simulink subsystem "ComputeState"  (R2020b)
settings: Solver=VariableStepAuto  StartTime=0.0  StopTime=10.0  RelTol=1e-3
libraries: simulink x2
settings Model: Creator=Marcus  LastModifiedBy=Marcus

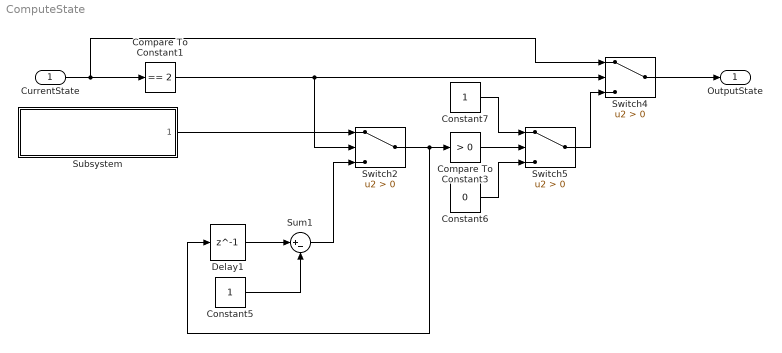
== system ComputeState ==
  CurrentState : Inport
  Compare To Constant1 : simulink/Logic and Bit Operations/Compare To Constant  relop===  const=2  OutDataTypeStr=boolean
  Compare To Constant3 : simulink/Logic and Bit Operations/Compare To Constant  relop=>  const=0  OutDataTypeStr=boolean
  Constant5 : Constant
  Constant6 : Constant  Value=0
  Constant7 : Constant
  Delay1 : Delay  DelayLength=1  InitialCondition=0
  Subsystem : Subsystem  ReferencedSubsystem=CyclesFromSeconds  sec=1
  Sum1 : Sum  Inputs=|+-
  Switch2 : Switch  Criteria=u2 > Threshold
  Switch4 : Switch  Criteria=u2 > Threshold
  Switch5 : Switch  Criteria=u2 > Threshold
  OutputState : Outport
  wires:
  Constant6/1 -> Switch5/3
  Switch2/1 -> Delay1/1, Compare To Constant3/1
  Compare To Constant1/1 -> Switch2/2, Switch4/2
  Switch5/1 -> Switch4/3
  Compare To Constant3/1 -> Switch5/2
  Sum1/1 -> Switch2/3
  Constant5/1 -> Sum1/2
  CurrentState/1 -> Compare To Constant1/1, Switch4/1
  Constant7/1 -> Switch5/1
  Delay1/1 -> Sum1/1
  Switch4/1 -> OutputState/1
  Subsystem/1 -> Switch2/1
